simulink model "scalar_kalman_ex_r2021a"  (R2021a)
settings: Solver=VariableStepAuto  StartTime=0.0  StopTime=22  RelTol=1e-3
libraries: simulink x2
settings Model: Creator=Daniel  LastModifiedBy=Daniel

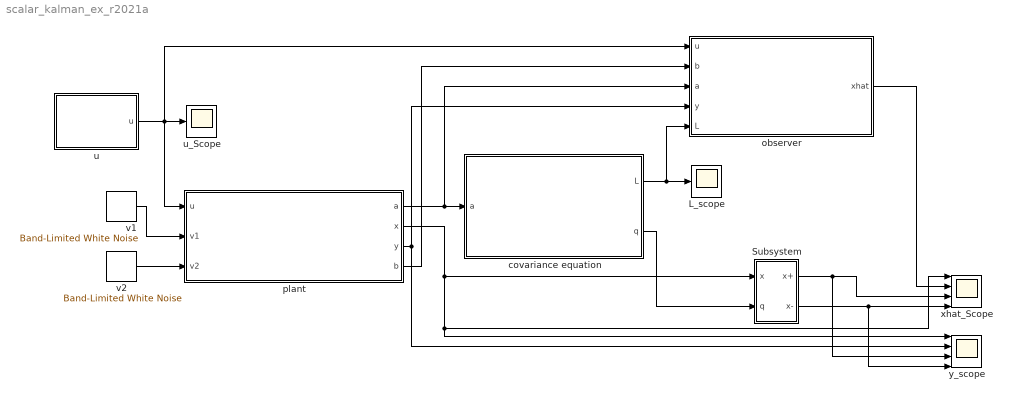
== system scalar_kalman_ex_r2021a ==
  L_scope : Scope
  Subsystem : Subsystem
  covariance equation : Subsystem
  observer : Subsystem
  plant : Subsystem
  u : Subsystem
  u_Scope : Scope
  v1 : simulink/Sources/Band-Limited White Noise  Cov=0.5^2*0.025  Ts=0.025  seed=[23341]
  v2 : simulink/Sources/Band-Limited White Noise  Cov=0.1^2*0.025  Ts=0.025  seed=[23341]
  xhat_Scope : Scope  NumInputPorts=4
  y_scope : Scope  NumInputPorts=4
  wires:
  observer/1(xhat) -> xhat_Scope/2
  plant/3(y) -> observer/4(y), y_scope/2
  plant/4(b) -> observer/2(b)
  u/1(u) -> plant/1(u), u_Scope/1, observer/1(u)
  v2/1 -> plant/3(v2)
  Subsystem/1(x+) -> y_scope/3, xhat_Scope/3
  v1/1 -> plant/2(v1)
  covariance equation/1(L) -> observer/5(L), L_scope/1
  covariance equation/2(q) -> Subsystem/2(q)
  plant/1(a) -> covariance equation/1(a), observer/3(a)
  plant/2(x) -> y_scope/1, xhat_Scope/1, Subsystem/1(x)
  Subsystem/2(x-) -> xhat_Scope/4, y_scope/4

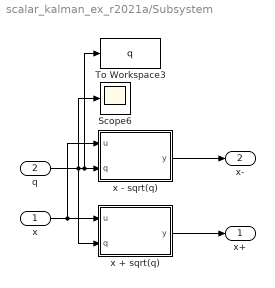
== system scalar_kalman_ex_r2021a/Subsystem ==
  x : Inport
  q : Inport  Port=2
  Scope6 : Scope
  To Workspace3 : ToWorkspace  VariableName=q  SaveFormat=Timeseries  SampleTime=-1
  x + sqrt(q) : MATLAB Function  TreatAsAtomicUnit=on
  x - sqrt(q) : MATLAB Function  TreatAsAtomicUnit=on
  x+ : Outport
  x- : Outport  Port=2
  wires:
  q/1 -> x - sqrt(q)/2(q), To Workspace3/1, Scope6/1, x + sqrt(q)/2(q)
  x/1 -> x + sqrt(q)/1(u), x - sqrt(q)/1(u)
  x - sqrt(q)/1(y) -> x-/1
  x + sqrt(q)/1(y) -> x+/1

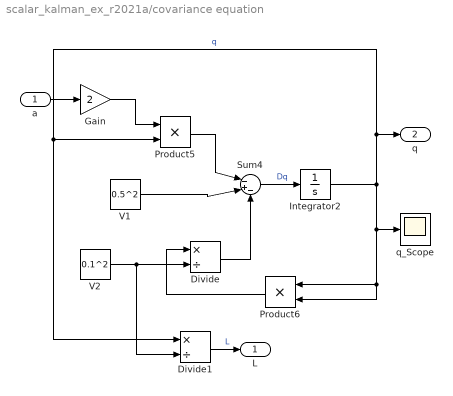
== system scalar_kalman_ex_r2021a/covariance equation ==
  a : Inport
  Divide : Product  Inputs=*/
  Divide1 : Product  Inputs=*/
  Gain : Gain  Gain=2
  Integrator2 : Integrator  InitialCondition=0.2
  Product5 : Product
  Product6 : Product
  Sum4 : Sum  Inputs=|-+-
  V1 : Constant  Value=0.5^2
  V2 : Constant  Value=0.1^2
  q_Scope : Scope
  L : Outport
  q : Outport  Port=2
  wires:
  Product6/1 -> Divide/1
  Divide1/1 -> L/1  "L"
  a/1 -> Gain/1
  Integrator2/1 -> q/1, Divide1/1, Product5/2, Product6/2, Product6/1, q_Scope/1  "q"
  V1/1 -> Sum4/2
  Product5/1 -> Sum4/1
  Divide/1 -> Sum4/3
  Sum4/1 -> Integrator2/1  "Dq"
  Gain/1 -> Product5/1
  V2/1 -> Divide1/2, Divide/2

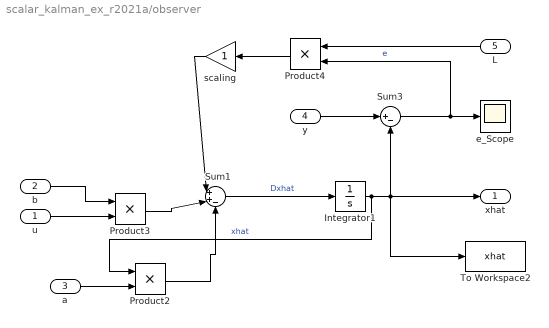
== system scalar_kalman_ex_r2021a/observer ==
  u : Inport
  b : Inport  Port=2
  a : Inport  Port=3
  y : Inport  Port=4
  L : Inport  Port=5
  Integrator1 : Integrator
  Product2 : Product
  Product3 : Product
  Product4 : Product
  Sum1 : Sum  Inputs=|++-
  Sum3 : Sum  Inputs=|+-
  To Workspace2 : ToWorkspace  VariableName=xhat  SaveFormat=Timeseries  SampleTime=-1
  e_Scope : Scope
  scaling : Gain
  xhat : Outport
  wires:
  Product2/1 -> Sum1/3
  b/1 -> Product3/1
  Sum1/1 -> Integrator1/1  "Dxhat"
  Product3/1 -> Sum1/2
  Product4/1 -> scaling/1
  scaling/1 -> Sum1/1
  L/1 -> Product4/1
  u/1 -> Product3/2
  y/1 -> Sum3/1
  a/1 -> Product2/2
  Sum3/1 -> Product4/2, e_Scope/1  "e"
  Integrator1/1 -> Sum3/2, To Workspace2/1, xhat/1, Product2/1  "xhat"

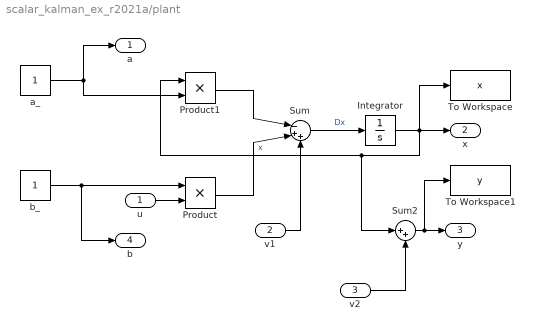
== system scalar_kalman_ex_r2021a/plant ==
  u : Inport
  v1 : Inport  Port=2
  v2 : Inport  Port=3
  Integrator : Integrator
  Product : Product
  Product1 : Product
  Sum : Sum  Inputs=|-++
  Sum2 : Sum  Inputs=|++
  To Workspace : ToWorkspace  VariableName=x  SaveFormat=Timeseries  SampleTime=-1
  To Workspace1 : ToWorkspace  VariableName=y  SaveFormat=Timeseries  SampleTime=-1
  a_ : Constant
  b_ : Constant
  a : Outport
  x : Outport  Port=2
  y : Outport  Port=3
  b : Outport  Port=4
  wires:
  Product1/1 -> Sum/1
  Integrator/1 -> To Workspace/1, Sum2/1, Product1/1, x/1  "x"
  Sum/1 -> Integrator/1  "Dx"
  Product/1 -> Sum/2
  b_/1 -> b/1, Product/1
  u/1 -> Product/2
  a_/1 -> Product1/2, a/1
  Sum2/1 -> To Workspace1/1, y/1
  v2/1 -> Sum2/2
  v1/1 -> Sum/3

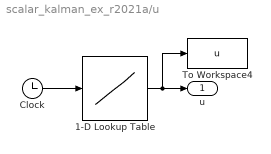
== system scalar_kalman_ex_r2021a/u ==
  1-D Lookup Table : Lookup_n-D  NumberOfTableDimensions=1  BreakpointsForDimension1=[0 5 10 15 22]'  Table=[0 1 -1 0 0]'  InterpMethod=Flat  InternalRulePriority=Speed  RndMeth=Simplest  InputSameDT=on
  Clock : Clock
  To Workspace4 : ToWorkspace  VariableName=u  SaveFormat=Timeseries  SampleTime=-1
  u : Outport
  wires:
  Clock/1 -> 1-D Lookup Table/1
  1-D Lookup Table/1 -> u/1, To Workspace4/1

== matlab function scalar_kalman_ex_r2021a/Subsystem/x + sqrt(q) ==
  data: u input; y output; q input
function y = fcn(u,q)

y = u + sqrt(q);

== matlab function scalar_kalman_ex_r2021a/Subsystem/x - sqrt(q) ==
  data: u input; y output; q input
function y = fcn(u,q)

y = u - sqrt(q);
